simulink library "actuator_library"  (R2018b)
settings: Solver=VariableStepAuto  StartTime=0.0  StopTime=10.0  RelTol=1e-3
undefined symbols (not defined in the file): MTQ_actuator_time, MTQ_DKE
libraries: simulink x3
settings Model: Creator=Andrea  LastModifiedBy=andrea

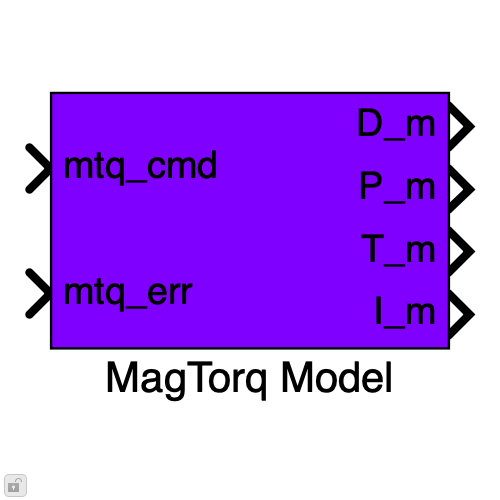
[thumbnail: Simulink's stored preview of the top-level diagram]
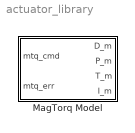
== system actuator_library ==
  MagTorq Model : Subsystem  mask(MagTorquers Model){mtq=MTQ_DKE, simstep=MTQ_actuator_time}
      mask prompts: mtq "Magnetorquers Data Structure"; simstep "Actuator Time (s)"
      mask help: © Andrea Colagrossi - Aerospace Science and Technology Dept. - PoliMi - 2018

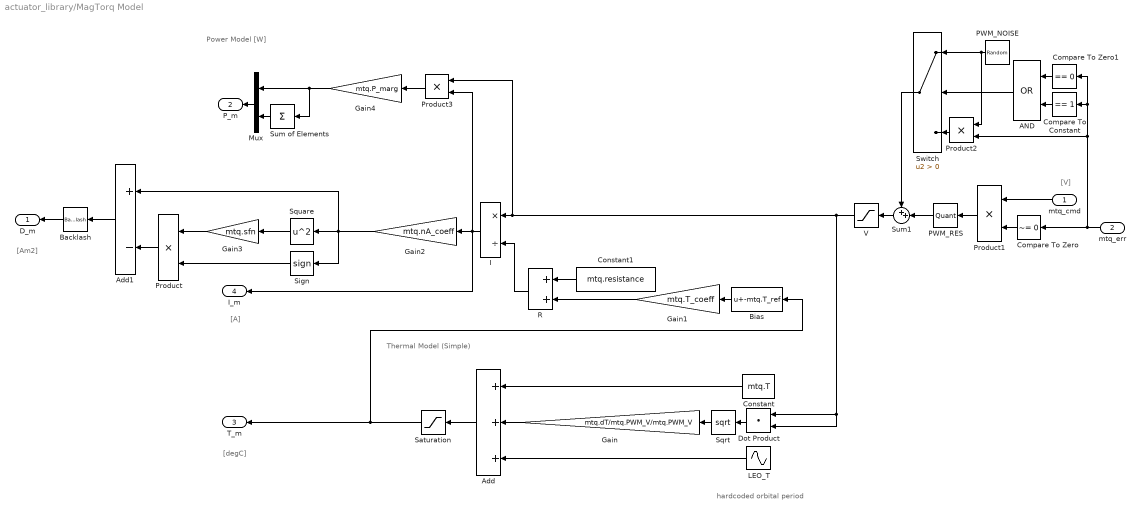
== system actuator_library/MagTorq Model ==
  note: [V]
  note: [Am2]
  note: [degC]
  note: Power Model [W]
  note: hardcoded orbital period
  note: Thermal Model (Simple)
  note: [A]
  mtq_cmd : Inport
  mtq_err : Inport  Port=2
  AND : Logic  Operator=OR  AllPortsSameDT=off  OutDataTypeStr=boolean
  Add : Sum  Inputs=+++
  Add1 : Sum  Inputs=+-
  Backlash : Backlash  BacklashWidth=2*mtq.residual
  Bias : Bias  Bias=-mtq.T_ref
  Compare To Constant : simulink/Logic and Bit Operations/Compare To Constant  relop===  const=1  OutDataTypeStr=boolean
  Compare To Zero : simulink/Logic and Bit Operations/Compare To Zero  relop=~=  OutDataTypeStr=boolean
  Compare To Zero1 : simulink/Logic and Bit Operations/Compare To Zero  relop===  OutDataTypeStr=boolean
  Constant : Constant  Value=mtq.T
  Constant1 : Constant  Value=mtq.resistance
  Dot Product : DotProduct  InputSameDT=on  OutDataTypeStr=Inherit: Inherit via internal rule
  Gain : Gain  Gain=mtq.dT/mtq.PWM_V/mtq.PWM_V
  Gain1 : Gain  Gain=mtq.T_coeff
  Gain2 : Gain  Gain=mtq.nA_coeff
  Gain3 : Gain  Gain=mtq.sfn
  Gain4 : Gain  Gain=mtq.P_marg
  I : Product  Inputs=*/
  LEO_T : Sin  Amplitude=mtq.dT  Frequency=2*pi/(1.5*3600)  SampleTime=simstep
  Mux : Mux  Inputs=2
  PWM_NOISE : RandomNumber  Mean=mtq.PWM_bias  Variance=mtq.PWM_noise.^2  Seed=mtq.PWM_noiseseed  SampleTime=simstep
  PWM_RES : Quantizer  QuantizationInterval=mtq.PWM_RES
  Product{,1..3} (4 alike) : Product
  R : Sum
  Saturation : Saturate  UpperLimit=mtq.T+mtq.dT  LowerLimit=-(mtq.T+mtq.dT)
  Sign : Signum
  Sqrt : Sqrt  SaturateOnIntegerOverflow=on
  Square : Math  Operator=square  SaturateOnIntegerOverflow=on
  Sum of Elements : Sum  Inputs=+
  Sum1 : Sum  Inputs=++|
  Switch : Switch  Criteria=u2 > Threshold
  V : Saturate  UpperLimit=mtq.PWM_V  LowerLimit=-mtq.PWM_V
  D_m : Outport  VectorParamsAs1DForOutWhenUnconnected=off
  P_m : Outport  Port=2  VectorParamsAs1DForOutWhenUnconnected=off
  T_m : Outport  Port=3  VectorParamsAs1DForOutWhenUnconnected=off
  I_m : Outport  Port=4  VectorParamsAs1DForOutWhenUnconnected=off
  wires:
  Saturation/1 -> T_m/1, Bias/1
  Product2/1 -> Switch/3
  Switch/1 -> Sum1/1
  PWM_NOISE/1 -> Switch/1, Product2/1
  mtq_err/1 -> Compare To Zero/1, Compare To Constant/1, Compare To Zero1/1, Product2/2
  AND/1 -> Switch/2
  Compare To Constant/1 -> AND/2
  Compare To Zero1/1 -> AND/1
  Compare To Zero/1 -> Product1/2
  Product1/1 -> PWM_RES/1
  mtq_cmd/1 -> Product1/1
  Gain4/1 -> Mux/1, Sum of Elements/1
  Sum of Elements/1 -> Mux/2
  Mux/1 -> P_m/1
  Product3/1 -> Gain4/1
  Backlash/1 -> D_m/1
  Sign/1 -> Product/2
  Product/1 -> Add1/2
  Add1/1 -> Backlash/1
  Square/1 -> Gain3/1
  Gain2/1 -> Sign/1, Square/1, Add1/1
  Gain3/1 -> Product/1
  I/1 -> Gain2/1, Product3/2, I_m/1
  V/1 -> I/1, Product3/1, Dot Product/2, Dot Product/1
  R/1 -> I/2
  Bias/1 -> Gain1/1
  Gain1/1 -> R/2
  Constant1/1 -> R/1
  Sum1/1 -> V/1
  PWM_RES/1 -> Sum1/2
  Add/1 -> Saturation/1
  LEO_T/1 -> Add/3
  Constant/1 -> Add/1
  Gain/1 -> Add/2
  Sqrt/1 -> Gain/1
  Dot Product/1 -> Sqrt/1
